simulink model "qpsk_ref"  (Simulink 7.9)
settings: Solver=FixedStepDiscrete  SolverMode=SingleTasking  StartTime=0.0  StopTime=1e4  RelTol=1e-3
PreLoadFcn:
  | qpsk_ref_init;
undefined symbols (not defined in the file or in its folder): get, qpsk_ref_params
libraries: commsink2 x6, commutil2 x2, commdigbbndpm3 x2, commfilt2 x2, commchan3 x1, dspsigops x1, commrandsrc2 x1
settings Model: Creator=sszilvasi  LastModifiedBy=sszilvasi
settings DataIOCC: SaveOutput=off  SignalLogging=off  SaveTime=off
settings OptimizationCC: InlineParams=on
settings DebuggingCC: AlgebraicLoopMsg=error

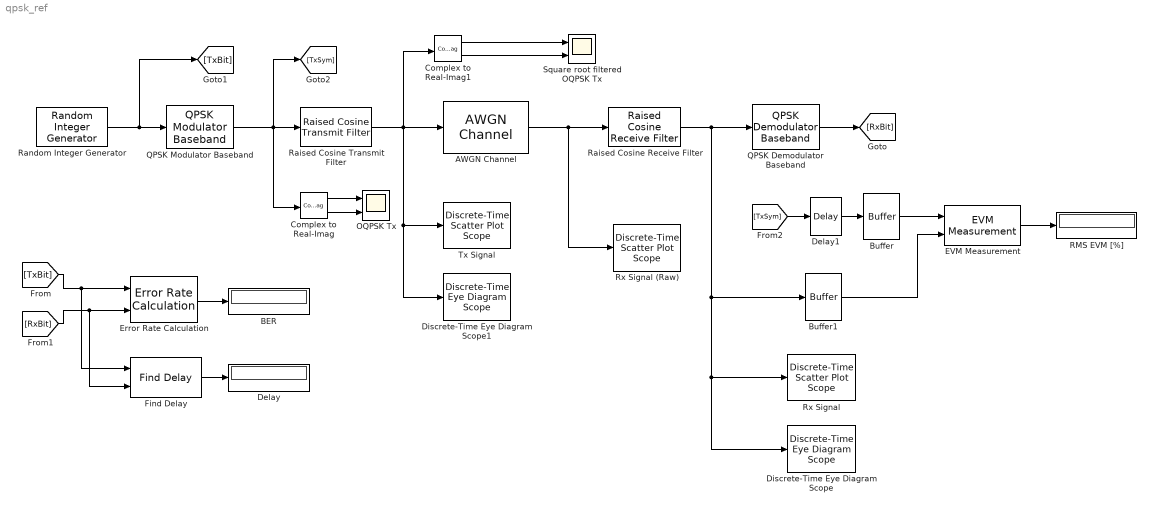
== system qpsk_ref ==
  AWGN Channel : commchan3/AWGN Channel  InputProcessing=Columns as channels (frame based)  seed=67  noiseMode="Signal to noise ratio  (SNR)"  EbNodB=30  EsNodB=10  SNRdB=qpsk_ref_params.snr  bitsPerSym=1  Ps=1  Tsym=1  variance=1
  BER : Display
  Buffer : Buffer  TreatMby1Signals=One channel
  Buffer1 : Buffer  TreatMby1Signals=One channel
  Complex to Real-Imag : ComplexToRealImag
  Complex to Real-Imag1 : ComplexToRealImag
  Delay : Display
  Delay1 : dspsigops/Delay  InputProcessing=Columns as channels (frame based)  dly_unit=Samples  delay=5  ic_detail=off  dif_ic_for_ch=off  dif_ic_for_dly=off  ic=0  reset_popup=None
  Discrete-Time Eye Diagram Scope : commsink2/Discrete-Time Eye Diagram Scope  Tag=EyeDiagram  sampPerSymb=16  offsetEye=0  symbPerTrace=1  numTraces=40  numNewFrames=10  LineStyles=-  LineColors=b  dupPoints=on  fading=on  render=on  AxisGrid=on  yMin=-1.42480746256597  yMax=1.48348317354032  inphaseLabel=In-phase Amplitude  quadratureLabel=Quadrature Amplitude  openScopeAtSimStart=off  dispDiagram=In-phase and Quadrature  FrameNumber=off  FigPos=get(0,'defaultfigureposition');  figTitle=Eye Diagram  block_type_=eye  numLinesMax=8
  Discrete-Time Eye Diagram Scope1 : commsink2/Discrete-Time Eye Diagram Scope  Tag=EyeDiagram  sampPerSymb=8  offsetEye=0  symbPerTrace=1  numTraces=40  numNewFrames=10  LineStyles=-  LineColors=b  dupPoints=on  fading=on  render=on  AxisGrid=on  yMin=-1.42480746256597  yMax=1.48348317354032  inphaseLabel=In-phase Amplitude  quadratureLabel=Quadrature Amplitude  openScopeAtSimStart=off  dispDiagram=In-phase and Quadrature  FrameNumber=off  FigPos=get(0,'defaultfigureposition');  figTitle=Eye Diagram  block_type_=eye  numLinesMax=8
  EVM Measurement : commutil2/EVM Measurement  normMethod=Average reference signal power  averagePower=1  peakPower=1  maxOrMinOut=off  percentileOut=off  percentileVal=95  nSym=off
  Error Rate Calculation : commsink2/Error Rate Calculation  N=qpsk_ref_params.N/2  st_delay=0  cp_mode=Entire frame  subframe=[]  PMode=Port  WsName=ErrorVec  RsMode2=off  stop=off  numErr=100  maxBits=1e6
  Find Delay : commutil2/Find Delay  corrLength=200  chgSigOP=off  stopUpdate=off  numConstDelay=3
  OQPSK Tx : Scope  NumInputPorts=2
      settings: YMin=-5~-5  YMax=5~5
  QPSK Demodulator Baseband : commdigbbndpm3/QPSK Demodulator Baseband  Ph=pi/4  Dec=Gray  OutType=Integer  DecType=Hard decision  VarSource=Dialog  Variance=1  outDtype1=Inherit via internal rule  outDtype2=Inherit via internal rule  derotateFactorWordLen=16
  QPSK Modulator Baseband : commdigbbndpm3/QPSK Modulator Baseband  InType=Integer  Enc=Gray  Ph=pi/4  outDtype=double  outWordLen=16  outUDDataType=sfix(16)  outFracLenMode=Best precision  outFracLen=15
  RMS EVM [%] : Display
  Raised Cosine Receive Filter : commfilt2/Raised Cosine Receive Filter  filtType=Square root  N=qpsk_ref_params.N  D=qpsk_ref_params.rc_group_delay  R=0.2  sampMode=Mute  saveAsFlag=0  rateMode=Downsampling  downFactor=qpsk_ref_params.N  downOffset=0  framing=Allow multirate processing  checkGain=Normalized  filterGain=1  checkCoeff=off  variableName=rcRxFilt  launchFVT=off  roundingMode=Floor  overflowMode=off
  Raised Cosine Transmit Filter : commfilt2/Raised Cosine Transmit Filter  filtType=Square root  D=qpsk_ref_params.rc_group_delay  R=0.2  sampMode=Mute  saveAsFlag=0  N=qpsk_ref_params.N  framing=Allow multirate processing  checkGain=Normalized  filterGain=1  checkCoeff=off  variableName=rcTxFilt  launchFVT=off  roundingMode=Floor  overflowMode=off
  Random Integer Generator : commrandsrc2/Random Integer Generator  mul=4  seed=37  Ts=1  frameBased=off  sampPerFrame=1  orient=off  outDataType=double
  Rx Signal : commsink2/Discrete-Time Scatter Plot Scope  Tag=ScatterPlot  sampPerSymb=16  offsetEye=0  numTraces=200  numNewFrames=40  LineMarkers=.  LineColors=b  fading=on  render=on  AxisGrid=on  xMin=-1  xMax=1  yMin=-1  yMax=1  inphaseLabel=In-phase Amplitude  quadratureLabel=Quadrature Amplitude  openScopeAtSimStart=off  FrameNumber=off  FigPos=get(0,'defaultfigureposition');  figTitle=Scatter Plot  numLinesMax=8  block_type_=scatter
  Rx Signal (Raw) : commsink2/Discrete-Time Scatter Plot Scope  Tag=ScatterPlot  sampPerSymb=16  offsetEye=0  numTraces=200  numNewFrames=40  LineMarkers=.  LineColors=b  fading=on  render=on  AxisGrid=on  xMin=-.5  xMax=.5  yMin=-.5  yMax=.5  inphaseLabel=In-phase Amplitude  quadratureLabel=Quadrature Amplitude  openScopeAtSimStart=off  FrameNumber=off  FigPos=get(0,'defaultfigureposition');  figTitle=Scatter Plot  numLinesMax=8  block_type_=scatter
  Square root filtered OQPSK Tx : Scope  NumInputPorts=2
      settings: YMin=-5~-5  YMax=5~5
  Tx Signal : commsink2/Discrete-Time Scatter Plot Scope  Tag=ScatterPlot  sampPerSymb=16  offsetEye=0  numTraces=200  numNewFrames=40  LineMarkers=.  LineColors=b  fading=on  render=on  AxisGrid=on  xMin=-.5  xMax=.5  yMin=-.5  yMax=.5  inphaseLabel=In-phase Amplitude  quadratureLabel=Quadrature Amplitude  openScopeAtSimStart=off  FrameNumber=off  FigPos=get(0,'defaultfigureposition');  figTitle=Scatter Plot  numLinesMax=8  block_type_=scatter
  wires:
  QPSK Modulator Baseband/1 -> [TxSym], Complex to Real-Imag/1, Raised Cosine Transmit Filter/1
  AWGN Channel/1 -> Raised Cosine Receive Filter/1, Rx Signal (Raw)/1
  Random Integer Generator/1 -> [TxBit], QPSK Modulator Baseband/1
  Raised Cosine Receive Filter/1 -> Buffer1/1, Discrete-Time Eye Diagram Scope/1, Rx Signal/1, QPSK Demodulator Baseband/1
  QPSK Demodulator Baseband/1 -> [RxBit]
  [TxBit] -> Error Rate Calculation/1, Find Delay/1
  [RxBit] -> Error Rate Calculation/2, Find Delay/2
  Error Rate Calculation/1 -> BER/1
  EVM Measurement/1 -> RMS EVM [%]/1
  Buffer1/1 -> EVM Measurement/2
  [TxSym] -> Delay1/1
  Delay1/1 -> Buffer/1
  Buffer/1 -> EVM Measurement/1
  Complex to Real-Imag/1 -> OQPSK Tx/1
  Complex to Real-Imag/2 -> OQPSK Tx/2
  Complex to Real-Imag1/1 -> Square root filtered OQPSK Tx/1
  Complex to Real-Imag1/2 -> Square root filtered OQPSK Tx/2
  Raised Cosine Transmit Filter/1 -> Tx Signal/1, Discrete-Time Eye Diagram Scope1/1, Complex to Real-Imag1/1, AWGN Channel/1
  Find Delay/1 -> Delay/1
